simulink model "TST_Rail_SetPointCor"  (R2016b)
settings: Solver=FixedStepDiscrete  StartTime=0.0  StopTime=simTime  FixedStep=sampleTime  RelTol=1e-3
values from neighbouring files (symbols this model uses):
  testCase = 1    [initTST_Rail_SetPointCor_001.m]
libraries: simulink x3, UnitTest_Lib x1
settings Model: Creator=zhengjinyan  LastModifiedBy=zhengjinyan
settings DebuggingCC: SignalRangeChecking=error

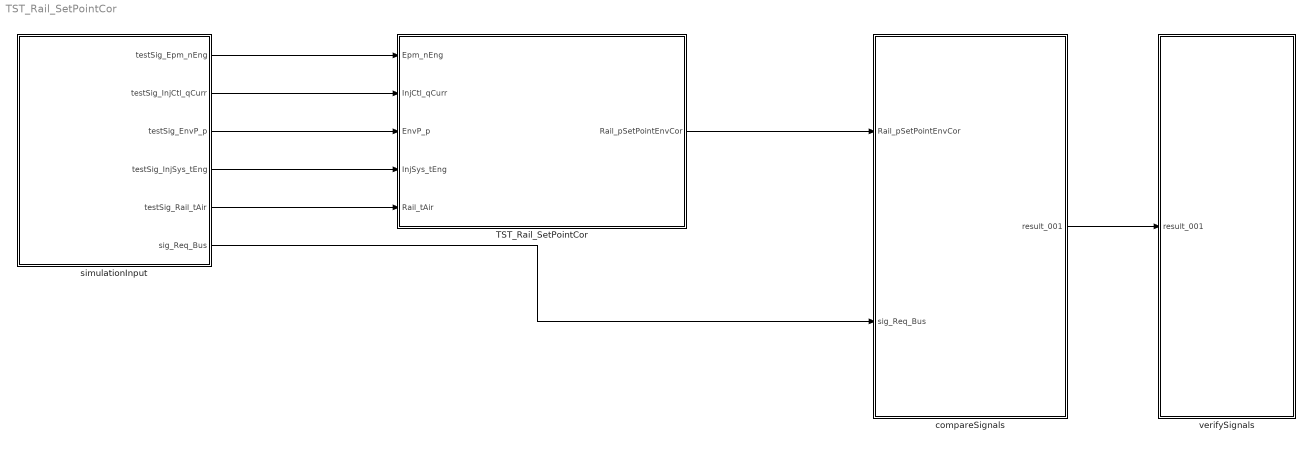
== system TST_Rail_SetPointCor ==
  TST_Rail_SetPointCor : Subsystem
  compareSignals : Subsystem
  simulationInput : Subsystem
  verifySignals : Subsystem
  wires:
  simulationInput/1(testSig_Epm_nEng) -> TST_Rail_SetPointCor/1(Epm_nEng)
  simulationInput/2(testSig_InjCtl_qCurr) -> TST_Rail_SetPointCor/2(InjCtl_qCurr)
  simulationInput/3(testSig_EnvP_p) -> TST_Rail_SetPointCor/3(EnvP_p)
  simulationInput/4(testSig_InjSys_tEng) -> TST_Rail_SetPointCor/4(InjSys_tEng)
  simulationInput/5(testSig_Rail_tAir) -> TST_Rail_SetPointCor/5(Rail_tAir)
  TST_Rail_SetPointCor/1(Rail_pSetPointEnvCor) -> compareSignals/1(Rail_pSetPointEnvCor)
  simulationInput/6(sig_Req_Bus) -> compareSignals/2(sig_Req_Bus)
  compareSignals/1(result_001) -> verifySignals/1(result_001)

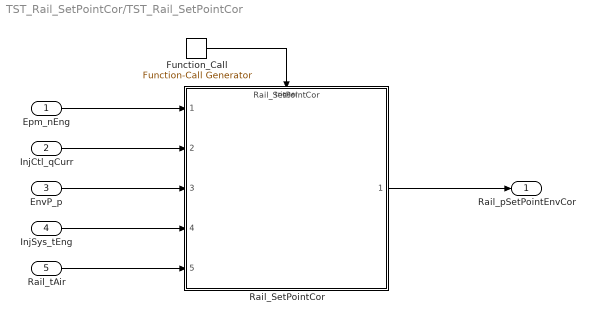
== system TST_Rail_SetPointCor/TST_Rail_SetPointCor ==
  Epm_nEng : Inport
  InjCtl_qCurr : Inport  Port=2
  EnvP_p : Inport  Port=3
  InjSys_tEng : Inport  Port=4
  Rail_tAir : Inport  Port=5
  Function_Call : simulink/Ports & Subsystems/Function-Call Generator  sample_time=sampleTime  numberOfIterations=1
  Rail_SetPointCor : ModelReference  ModelNameDialog=Rail_SetPointCor  SimulationMode=Normal  ModelReferenceVersion=1.16  TriggerPortName=function  TriggerPortTriggerType=function-call  TriggerPortStatesWhenEnabling=held
  Rail_pSetPointEnvCor : Outport
  wires:
  Function_Call/1 -> Rail_SetPointCor/Trigger
  Epm_nEng/1 -> Rail_SetPointCor/1
  InjCtl_qCurr/1 -> Rail_SetPointCor/2
  EnvP_p/1 -> Rail_SetPointCor/3
  InjSys_tEng/1 -> Rail_SetPointCor/4
  Rail_tAir/1 -> Rail_SetPointCor/5
  Rail_SetPointCor/1 -> Rail_pSetPointEnvCor/1

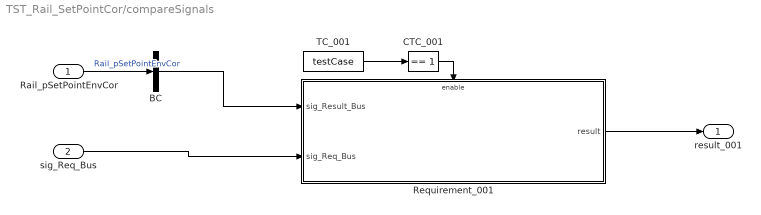
== system TST_Rail_SetPointCor/compareSignals ==
  Rail_pSetPointEnvCor : Inport
  sig_Req_Bus : Inport  Port=2
  BC : BusCreator  Inputs=1
  CTC_001 : simulink/Logic and Bit Operations/Compare To Constant  relop===  const=1  OutDataTypeStr=boolean
  Requirement_001 : Subsystem
  TC_001 : Constant  Value=testCase
  result_001 : Outport
  wires:
  Rail_pSetPointEnvCor/1 -> BC/1  "Rail_pSetPointEnvCor"
  TC_001/1 -> CTC_001/1
  CTC_001/1 -> Requirement_001/Enable
  sig_Req_Bus/1 -> Requirement_001/2(sig_Req_Bus)
  BC/1 -> Requirement_001/1(sig_Result_Bus)
  Requirement_001/1(result) -> result_001/1

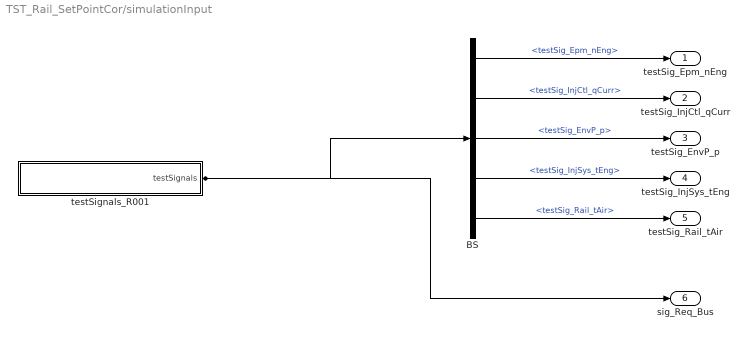
== system TST_Rail_SetPointCor/simulationInput ==
  BS : BusSelector  OutputSignals=testSig_Epm_nEng,testSig_InjCtl_qCurr,testSig_EnvP_p,testSig_InjSys_tEng,testSig_Rail_tAir
  testSignals_R001 : Subsystem
  testSig_Epm_nEng : Outport
  testSig_InjCtl_qCurr : Outport  Port=2
  testSig_EnvP_p : Outport  Port=3
  testSig_InjSys_tEng : Outport  Port=4
  testSig_Rail_tAir : Outport  Port=5
  sig_Req_Bus : Outport  Port=6
  wires:
  BS/1 -> testSig_Epm_nEng/1  "<testSig_Epm_nEng>"
  BS/2 -> testSig_InjCtl_qCurr/1  "<testSig_InjCtl_qCurr>"
  BS/3 -> testSig_EnvP_p/1  "<testSig_EnvP_p>"
  BS/4 -> testSig_InjSys_tEng/1  "<testSig_InjSys_tEng>"
  BS/5 -> testSig_Rail_tAir/1  "<testSig_Rail_tAir>"
  testSignals_R001/1(testSignals) -> BS/1, sig_Req_Bus/1

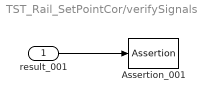
== system TST_Rail_SetPointCor/verifySignals ==
  result_001 : Inport
  Assertion_001 : Assertion  Enabled=off
  wires:
  result_001/1 -> Assertion_001/1

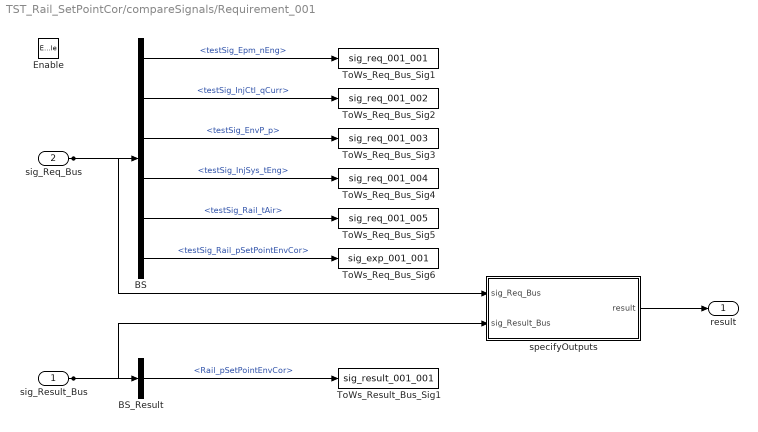
== system TST_Rail_SetPointCor/compareSignals/Requirement_001 ==
  sig_Result_Bus : Inport
  sig_Req_Bus : Inport  Port=2
  Enable : EnablePort
  BS : BusSelector  OutputSignals=testSig_Epm_nEng,testSig_InjCtl_qCurr,testSig_EnvP_p,testSig_InjSys_tEng,testSig_Rail_tAir,testSig_Rail_pSetPointEnvCor
  BS_Result : BusSelector  OutputSignals=Rail_pSetPointEnvCor
  ToWs_Req_Bus_Sig1 : ToWorkspace  VariableName=sig_req_001_001  SaveFormat=Structure With Time
  ToWs_Req_Bus_Sig2 : ToWorkspace  VariableName=sig_req_001_002  SaveFormat=Structure With Time
  ToWs_Req_Bus_Sig3 : ToWorkspace  VariableName=sig_req_001_003  SaveFormat=Structure With Time
  ToWs_Req_Bus_Sig4 : ToWorkspace  VariableName=sig_req_001_004  SaveFormat=Structure With Time
  ToWs_Req_Bus_Sig5 : ToWorkspace  VariableName=sig_req_001_005  SaveFormat=Structure With Time
  ToWs_Req_Bus_Sig6 : ToWorkspace  VariableName=sig_exp_001_001  SaveFormat=Structure With Time
  ToWs_Result_Bus_Sig1 : ToWorkspace  VariableName=sig_result_001_001  SaveFormat=Structure With Time
  specifyOutputs : Subsystem
  result : Outport
  wires:
  sig_Req_Bus/1 -> BS/1, specifyOutputs/1(sig_Req_Bus)
  BS/1 -> ToWs_Req_Bus_Sig1/1  "<testSig_Epm_nEng>"
  BS/2 -> ToWs_Req_Bus_Sig2/1  "<testSig_InjCtl_qCurr>"
  BS/3 -> ToWs_Req_Bus_Sig3/1  "<testSig_EnvP_p>"
  BS/4 -> ToWs_Req_Bus_Sig4/1  "<testSig_InjSys_tEng>"
  BS/5 -> ToWs_Req_Bus_Sig5/1  "<testSig_Rail_tAir>"
  BS/6 -> ToWs_Req_Bus_Sig6/1  "<testSig_Rail_pSetPointEnvCor>"
  sig_Result_Bus/1 -> BS_Result/1, specifyOutputs/2(sig_Result_Bus)
  BS_Result/1 -> ToWs_Result_Bus_Sig1/1  "<Rail_pSetPointEnvCor>"
  specifyOutputs/1(result) -> result/1

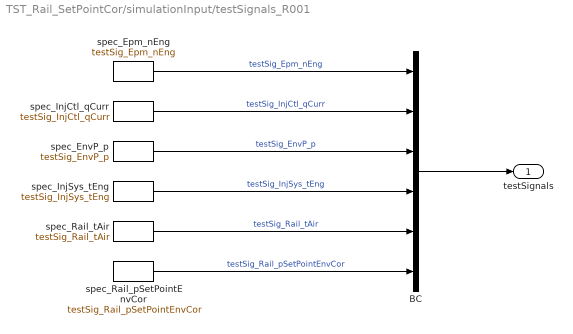
== system TST_Rail_SetPointCor/simulationInput/testSignals_R001 ==
  BC : BusCreator  Inputs=6
  spec_EnvP_p : FromWorkspace  VariableName=testSig_EnvP_p  Interpolate=off  OutputAfterFinalValue=Holding final value
  spec_Epm_nEng : FromWorkspace  VariableName=testSig_Epm_nEng  Interpolate=off  OutputAfterFinalValue=Holding final value
  spec_InjCtl_qCurr : FromWorkspace  VariableName=testSig_InjCtl_qCurr  Interpolate=off  OutputAfterFinalValue=Holding final value
  spec_InjSys_tEng : FromWorkspace  VariableName=testSig_InjSys_tEng  Interpolate=off  OutputAfterFinalValue=Holding final value
  spec_Rail_pSetPointEnvCor : FromWorkspace  VariableName=testSig_Rail_pSetPointEnvCor  Interpolate=off  OutputAfterFinalValue=Holding final value
  spec_Rail_tAir : FromWorkspace  VariableName=testSig_Rail_tAir  Interpolate=off  OutputAfterFinalValue=Holding final value
  testSignals : Outport
  wires:
  BC/1 -> testSignals/1
  spec_Epm_nEng/1 -> BC/1  "testSig_Epm_nEng"
  spec_InjCtl_qCurr/1 -> BC/2  "testSig_InjCtl_qCurr"
  spec_EnvP_p/1 -> BC/3  "testSig_EnvP_p"
  spec_InjSys_tEng/1 -> BC/4  "testSig_InjSys_tEng"
  spec_Rail_tAir/1 -> BC/5  "testSig_Rail_tAir"
  spec_Rail_pSetPointEnvCor/1 -> BC/6  "testSig_Rail_pSetPointEnvCor"

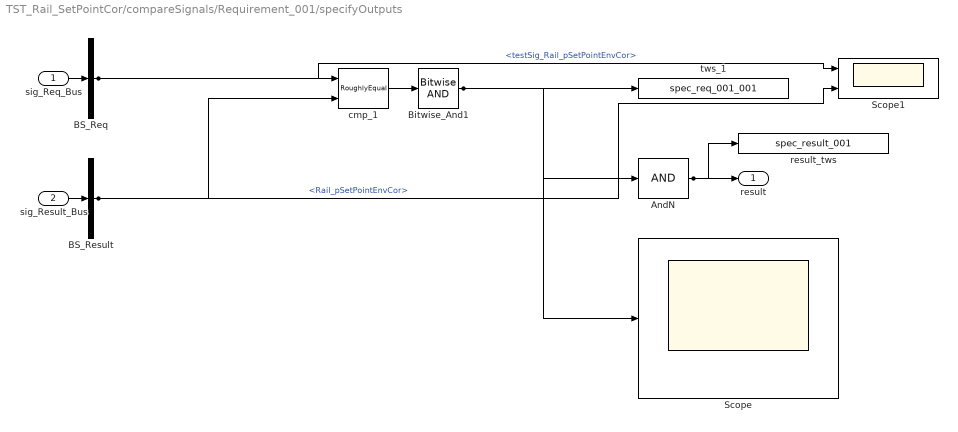
== system TST_Rail_SetPointCor/compareSignals/Requirement_001/specifyOutputs ==
  sig_Req_Bus : Inport
  sig_Result_Bus : Inport  Port=2
  AndN : Logic  Inputs=1
  BS_Req : BusSelector  OutputSignals=testSig_Rail_pSetPointEnvCor
  BS_Result : BusSelector  OutputSignals=Rail_pSetPointEnvCor
  Bitwise_And1 : simulink/Logic and Bit Operations/Bitwise Operator  logicop=AND  UseBitMask=off  BitMask=bin2dec('11011001')  BitMaskRealWorld=Stored Integer
  Scope : Scope
  Scope1 : Scope  NumInputPorts=2
  cmp_1 : UnitTest_Lib/RoughlyEqual  slope=0.1
  result_tws : ToWorkspace  VariableName=spec_result_001
  tws_1 : ToWorkspace  VariableName=spec_req_001_001
  result : Outport
  wires:
  sig_Req_Bus/1 -> BS_Req/1
  sig_Result_Bus/1 -> BS_Result/1
  AndN/1 -> result/1, result_tws/1
  BS_Req/1 -> cmp_1/1, Scope1/1  "<testSig_Rail_pSetPointEnvCor>"
  BS_Result/1 -> cmp_1/2, Scope1/2  "<Rail_pSetPointEnvCor>"
  cmp_1/1 -> Bitwise_And1/1
  Bitwise_And1/1 -> tws_1/1, AndN/1, Scope/1
